simulink model "sampleModel166"  (R2021b)
settings: Solver=VariableStepAuto  StartTime=0.0  StopTime=10.0  RelTol=1e-3
settings Model: Creator=user  LastModifiedBy=user

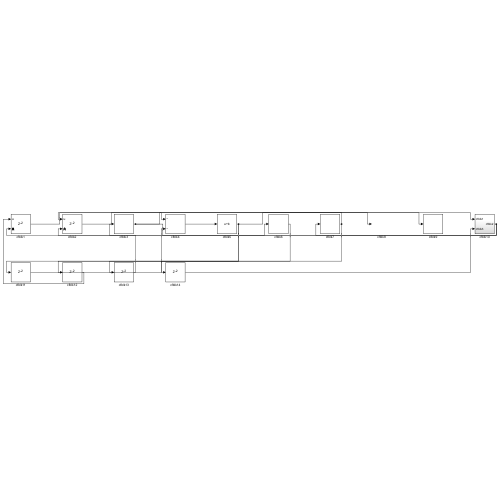
[thumbnail: Simulink's stored preview of the top-level diagram]
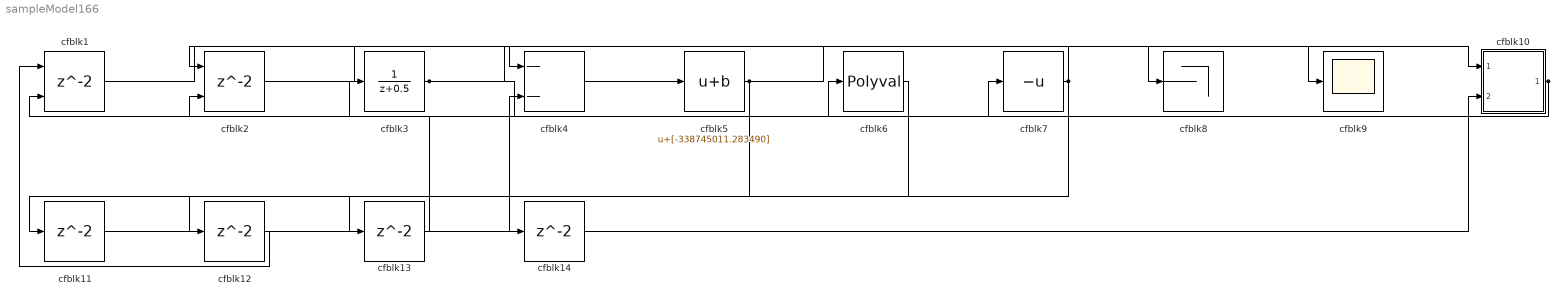
== system sampleModel166 ==
  cfblk1 : Delay  ShowEnablePort=on  SampleTime=1
      settings: InputPortMap=u0,e6
  cfblk10 : Subsystem
  cfblk{11..14} (4 alike) : Delay  SampleTime=1
  cfblk2 : Delay  ShowEnablePort=on  SampleTime=1
      settings: InputPortMap=u0,e6
  cfblk3 : DiscreteTransferFcn  SampleTime=1
  cfblk4 : Sum  Inputs=--
  cfblk5 : Bias  Bias=[-338745011.283490]
  cfblk6 : Polyval  Coefs=[ +2.081618890e-019, -1.441693666e-014, +4.719686976e-010, -8.536869453e-006, +1.621573104e-001, -8.087801117e+001 ]
  cfblk7 : UnaryMinus
  cfblk8 : Terminator
  cfblk9 : Scope
  wires:
  cfblk2/1 -> cfblk9/1
  cfblk3/1 -> cfblk6/1, cfblk10/1(cfblk1)
  cfblk4/1 -> cfblk5/1
  cfblk10/1(cfblk2) -> cfblk7/1, cfblk2/2, cfblk1/2
  cfblk1/1 -> cfblk4/1
  cfblk7/1 -> cfblk2/1, cfblk14/1
  cfblk5/1 -> cfblk8/1, cfblk11/1, cfblk12/1
  cfblk11/1 -> cfblk4/2
  cfblk12/1 -> cfblk1/1
  cfblk6/1 -> cfblk13/1
  cfblk13/1 -> cfblk3/1
  cfblk14/1 -> cfblk10/2(cfblk3)

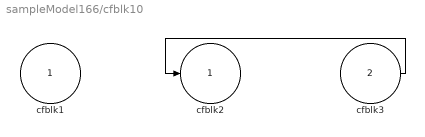
== system sampleModel166/cfblk10 ==
  cfblk1 : Inport
  cfblk3 : Inport  Port=2
  cfblk2 : Outport
  wires:
  cfblk3/1 -> cfblk2/1
